simulink model "SuR_Projekt_Wegpunkt_v3"  (R2023a)
settings: Solver=FixedStepDiscrete  StartTime=0.0  StopTime=inf  FixedStep=0.1  RelTol=1e-3  EnableMultiTasking=on
libraries: quarc_library x6
settings Model: ExtModeTrigDuration=10000  Creator=Student  LastModifiedBy=Student
settings SolverCC: AlgebraicLoopSolver=TrustRegion  PositivePriorityOrder=on
settings DataIOCC: ReturnWorkspaceOutputs=off
settings DebuggingCC: UnconnectedInputMsg=warning  UnconnectedOutputMsg=warning  UnconnectedLineMsg=warning  ArithmeticOperatorsInVariantConditions=warning
settings ModelReferenceCC: EnableRefExpFcnMdlSchedulingChecks=on
settings SFSimCC: SimUseLocalCustomCode=off  CustomCodeUndefinedFunction=UseInterfaceOnly
settings RTWCC: Description=QUARC Win64 Target Using Toolchain  SystemTargetFile=quarc_win64.tlc  TemplateMakefile=quarc_default_tmf  RTWUseLocalCustomCode=off  Toolchain=QUARC win64 | nmake (64-bit Windows)  BuildConfiguration=Faster Runs
settings CodeAppCC: StateflowObjectComments=on
settings STFCustomTargetCC: SystemTargetFile=quarc_win64.tlc
settings GRTTargetCC: ParMdlRefBuildCompliant=off  CompOptLevelCompliant=off  CombineOutputUpdateFcns=off  MatFileLogging=off  CPPClassGenCompliant=off  GRTInterface=on  ExtMode=on  ExtModeMexFile=quarc_comm
settings ConfigComp: CovMetricSettings=dswe

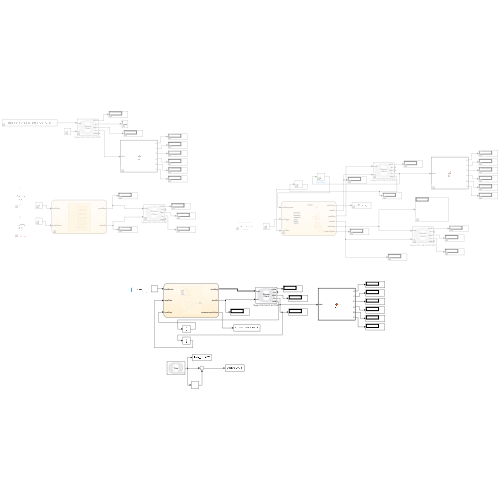
[thumbnail: Simulink's stored preview of the top-level diagram]
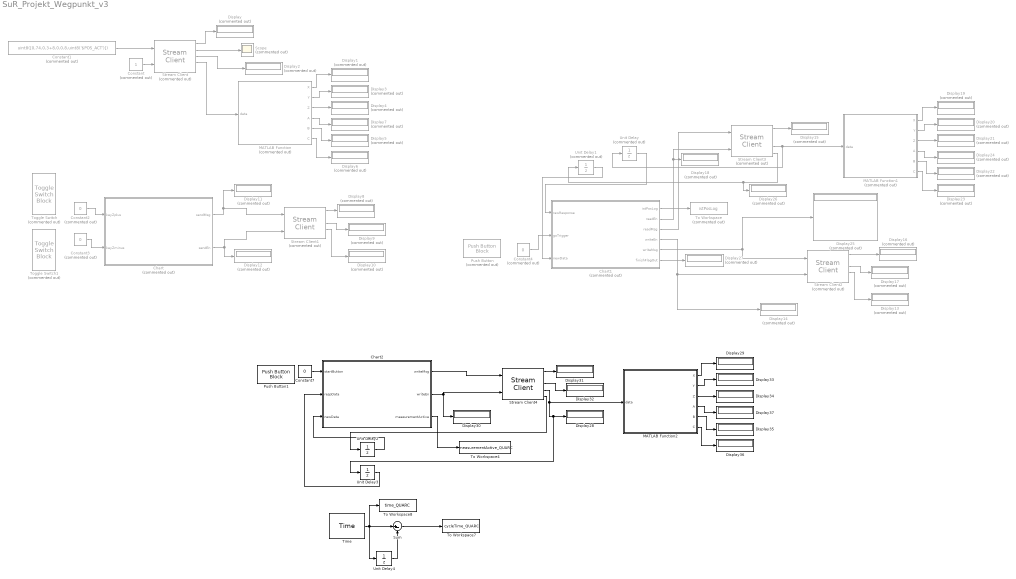
== system SuR_Projekt_Wegpunkt_v3 ==
  Chart : Stateflow chart  Commented=on  TreatAsAtomicUnit=on
  Chart1 : Stateflow chart  Commented=on  TreatAsAtomicUnit=on
  Chart2 : Stateflow chart  TreatAsAtomicUnit=on
  Constant : Constant  Commented=on
  Constant1 : Constant  Commented=on  Value=uint8([0,74,0,3+8,0,0,8,uint8('$POS_ACT')])  OutDataTypeStr=uint8
  Constant2 : Constant  Commented=on  Value=0  OutDataTypeStr=boolean
  Constant3 : Constant  Commented=on  Value=0  OutDataTypeStr=boolean
  Constant4 : Constant  Commented=on  Value=0  OutDataTypeStr=boolean
  Constant7 : Constant  Value=0
  Display{,1..27} (28 alike) : Display  Commented=on
  Display{28..37} (10 alike) : Display
  MATLAB Function : MATLAB Function  Commented=on  TreatAsAtomicUnit=on
  MATLAB Function1 : MATLAB Function  Commented=on  TreatAsAtomicUnit=on
  MATLAB Function2 : MATLAB Function  TreatAsAtomicUnit=on
  Push Button : PushButtonBlock  Commented=on  OffValue=0.000000
  Push Button1 : PushButtonBlock  OffValue=0.000000
  Scope : Scope  Commented=on
  Stream Client : quarc_library/Communications/Basic/Stream Client  Commented=on  uri_source=Specify via dialog (do not evaluate)  uri=tcpip://192.168.41.64:7000  send_buffer_size=1460  receive_buffer_size=1460  byte_order=little endian (Intel - LSB first)  optimization=Minimum latency  send_options=Send all data  receive_options=Receive all data  default_value=[uint8(0);uint8(0);uint8(0);uint8(0);uint8(0);uint8(0);uint8(0);uint8(0);uint8(0);uint8(0);uint8(0);uint8(0);uint8(0);uint8(0);uint8(0);uint8(0);uint8(0);uint8(0);uint8(0);uint8(0);uint8(0);uint8(0);uint8(0);uint8(0);uint8(0);uint8(0);uint8(0);uint8(0);uint8(0);uint8(0);uint8(0);uint8(0);uint8(0);uint8(0);uint8(0);uint8(0);uint8(0);uint8(0);uint8(0);uint8(0);uint8(0);uint8(0);uint8(0);uint8(0);uint8(0);uint8(0);uint8(0);uint8(0);uint8(0);uint8(0);uint8(0);uint8(0);uint8(0);uint8(0);uint8(0);uint8(0);uint8(0);uint8(0);uint8(0);uint8(0);uint8(0);uint8(0);uint8(0);uint8(0);uint8(0);uint8(0);uint8(0);uint8(0);uint8(0);uint8(0);uint8(0);uint8(0);uint8(0);uint8(0);uint8(0);uint8(0);uint8(0);uint8(0);uint8(0);uint8(0);uint8(0);uint8(0);uint8(0);uint8(0);uint8(0);uint8(0);uint8(0);uint8(0);uint8(0);uint8(0);uint8(0);uint8(0);uint8(0);uint8(0);uint8(0);uint8(0);uint8(0);uint8(0);uint8(0);uint8(0);uint8(0);uint8(0);uint8(0);uint8(0);uint8(0);uint8(0);uint8(0);uint8(0);uint8(0);uint8(0);uint8(0);uint8(0);uint8(0);uint8(0);uint8(0);uint8(0);uint8(0);uint8(0);uint8(0);uint8(0);uint8(0);uint8(0);uint8(0);uint8(0);uint8(0);uint8(0);uint8(0);uint8(0);uint8(0);uint8(0);uint8(0);uint8(0);uint8(0);uint8(0);uint8(0);uint8(0);uint8(0);uint8(0);uint8(0);uint8(0);uint8(0);uint8(0);uint8(0);uint8(0);uint8(0);uint8(0);uint8(0);uint8(0);uint8(0);uint8(0);uint8(0);uint8(0);uint8(0);uint8(0);uint8(0);uint8(0);uint8(0);uint8(0);uint8(0);uint8(0);uint8(0);uint8(0);uint8(0);uint8(0);uint8(0);uint8(0);uint8(0);uint8(0);uint8(0);uint8(0);uint8(0);uint8(0);uint8(0);uint8(0);uint8(0);uint8(0);uint8(0);uint8(0);uint8(0);uint8(0);uint8(0);uint8(0);uint8(0);uint8(0);uint8(0);uint8(0);uint8(0);uint8(0);uint8(0);uint8(0);uint8(0);uint8(0);uint8(0);uint8(0);uint8(0);uint8(0);uint8(0);uint8(0);uint8(0);uint8(0);uint8(0);uint8(0);uint8(0);uint8(0);uint8(0);uint8(0);uint8(0);uint8(0);uint8(0);uint8(0);uint8(0);uint8(0);uint8(0);uint8(0);uint8(0);uint8(0);uint8(0);uint8(0);uint8(0);uint8(0);uint8(0);uint8(0);uint8(0);uint8(0);uint8(0);uint8(0);uint8(0);uint8(0);uint8(0);uint8(0);uint8(0);uint8(0);uint8(0);uint8(0);uint8(0);uint8(0);uint8(0);uint8(0);uint8(0);uint8(0);uint8(0);uint8(0);uint8(0);uint8(0);uint8(0);uint8(0);uint8(0);uint8(0);uint8(0);uint8(0);uint8(0);uint8(0);uint8(0);uint8(0);uint8(0);uint8(0)]  sample_time=qc_get_step_size  active=off  implementation=Use blocking I/O in a separate thread  send_fifo_size=1000  receive_fifo_size=1000  send_priority=0  receive_priority=0  send_dimensions=off  receive_dimensions=off  max_dimensions=-1  data_type=uint8  type_expr=BusObject
      settings: AttributesFormatString="\"tcpip://192.168.41.64:7000\""
  Stream Client1 : quarc_library/Communications/Basic/Stream Client  Commented=on  uri_source=Specify via dialog (do not evaluate)  uri=tcpip://192.168.41.64:7000  send_buffer_size=1460  receive_buffer_size=1460  byte_order=little endian (Intel - LSB first)  optimization=Minimum latency  send_options=Send all data  receive_options=Receive all data  default_value=zeros(256,1,'uint8')  sample_time=qc_get_step_size  active=off  implementation=Use blocking I/O in a separate thread  send_fifo_size=1000  receive_fifo_size=1000  send_priority=0  receive_priority=0  send_dimensions=off  receive_dimensions=off  max_dimensions=-1  data_type=uint8  type_expr=BusObject
      settings: AttributesFormatString="\"tcpip://192.168.41.64:7000\""
  Stream Client2 : quarc_library/Communications/Basic/Stream Client  Commented=on  uri_source=Specify via dialog (do not evaluate)  uri=tcpip://192.168.41.64:7000  send_buffer_size=1460  receive_buffer_size=1460  byte_order=little endian (Intel - LSB first)  optimization=Minimum latency  send_options=Send all data  receive_options=Receive all data  default_value=zeros(256,1,'uint8')  sample_time=qc_get_step_size  active=off  implementation=Use blocking I/O in a separate thread  send_fifo_size=1000  receive_fifo_size=1000  send_priority=0  receive_priority=0  send_dimensions=off  receive_dimensions=off  max_dimensions=-1  data_type=uint8  type_expr=BusObject
      settings: AttributesFormatString="\"tcpip://192.168.41.64:7000\""
  Stream Client3 : quarc_library/Communications/Basic/Stream Client  Commented=on  uri_source=Specify via dialog (do not evaluate)  uri=tcpip://192.168.41.64:7000  send_buffer_size=1460  receive_buffer_size=1460  byte_order=little endian (Intel - LSB first)  optimization=Minimum latency  send_options=Send all data  receive_options=Receive all data  default_value=zeros(256,1,'uint8')  sample_time=qc_get_step_size  active=off  implementation=Use blocking I/O in a separate thread  send_fifo_size=1000  receive_fifo_size=1000  send_priority=0  receive_priority=0  send_dimensions=off  receive_dimensions=off  max_dimensions=-1  data_type=uint8  type_expr=BusObject
      settings: AttributesFormatString="\"tcpip://192.168.41.64:7000\""
  Stream Client4 : quarc_library/Communications/Basic/Stream Client  uri_source=Specify via dialog (do not evaluate)  uri=tcpip://192.168.41.64:7000  send_buffer_size=1460  receive_buffer_size=1460  byte_order=little endian (Intel - LSB first)  optimization=Minimum latency  send_options=Send all data  receive_options=Receive all data  default_value=zeros(256,1,'uint8')  sample_time=qc_get_step_size  active=off  implementation=Use blocking I/O in a separate thread  send_fifo_size=1000  receive_fifo_size=1000  send_priority=0  receive_priority=0  send_dimensions=off  receive_dimensions=off  max_dimensions=-1  data_type=uint8  type_expr=BusObject
      settings: AttributesFormatString="\"tcpip://192.168.41.64:7000\""
  Sum : Sum  Inputs=|+-
  Time : quarc_library/Sources/Time/Time  time_source=Wall clock  sample_time=qc_get_step_size
  To Workspace : ToWorkspace  Commented=on  VariableName=istPosLog  SampleTime=-1
  To Workspace4 : ToWorkspace  VariableName=measurementActive_QUARC  SaveFormat=Structure With Time  SampleTime=-1
  To Workspace7 : ToWorkspace  VariableName=cycleTime_QUARC  SaveFormat=Structure With Time  SampleTime=-1
  To Workspace8 : ToWorkspace  VariableName=time_QUARC  SaveFormat=Structure With Time  SampleTime=-1
  Toggle Switch : ToggleSwitchBlock  Commented=on
      settings: Values={{'Off', 'On'}, [0 1]}
  Toggle Switch1 : ToggleSwitchBlock  Commented=on
      settings: Values={{'Off', 'On'}, [0 1]}
  Unit Delay : UnitDelay  Commented=on  InitialCondition=uint8(zeros(1,256))  SampleTime=-1  HasFrameUpgradeWarning=on
  Unit Delay1 : UnitDelay  Commented=on  InitialCondition=uint8(zeros(1,1))  SampleTime=-1  HasFrameUpgradeWarning=on
  Unit Delay2 : UnitDelay  InitialCondition=uint8(zeros(1,1))  SampleTime=-1  HasFrameUpgradeWarning=on
  Unit Delay3 : UnitDelay  InitialCondition=uint8(zeros(1,256))  SampleTime=-1  HasFrameUpgradeWarning=on
  Unit Delay4 : UnitDelay  SampleTime=-1  HasFrameUpgradeWarning=on
  wires:
  Stream Client/1 -> Display/1
  Stream Client/2 -> Scope/1
  Constant1/1 -> Stream Client/1
  Stream Client/4 -> MATLAB Function/1(data)
  Stream Client/3 -> Display2/1
  MATLAB Function/1(X) -> Display1/1
  MATLAB Function/2(Y) -> Display3/1
  MATLAB Function/3(Z) -> Display4/1
  MATLAB Function/4(A) -> Display7/1
  MATLAB Function/5(B) -> Display5/1
  MATLAB Function/6(C) -> Display6/1
  Stream Client1/1 -> Display8/1
  Constant/1 -> Stream Client/2
  Chart/1(sendMsg) -> Display11/1, Stream Client1/1
  Chart/2(sendEn) -> Stream Client1/2, Display12/1
  Constant3/1 -> Chart/2(keyZminus)
  Stream Client1/3 -> Display9/1
  Stream Client1/4 -> Display10/1
  Constant2/1 -> Chart/1(keyZplus)
  Stream Client2/4 -> Display13/1
  Stream Client2/1 -> Display16/1
  Stream Client2/3 -> Display17/1
  Constant4/1 -> Chart1/2(goTrigger)
  Chart1/5(writeMsg) -> Stream Client2/1, Display25/1
  Chart1/4(writeEn) -> Display14/1, Stream Client2/2
  Chart1/3(readMsg) -> Stream Client3/1
  Chart1/2(readEn) -> Stream Client3/2, Display18/1
  Chart1/1(istPosLog) -> To Workspace/1
  Stream Client3/1 -> Display15/1
  Stream Client3/4 -> MATLAB Function1/1(data), Unit Delay/1
  Unit Delay/1 -> Chart1/1(rawResponse)
  MATLAB Function1/4(A) -> Display24/1
  MATLAB Function1/6(C) -> Display23/1
  MATLAB Function1/3(Z) -> Display21/1
  MATLAB Function1/2(Y) -> Display20/1
  MATLAB Function1/5(B) -> Display22/1
  MATLAB Function1/1(X) -> Display19/1
  Chart1/6(finishFlagOut) -> Display27/1
  Unit Delay1/1 -> Chart1/3(newData)
  Stream Client3/5 -> Display26/1, Unit Delay1/1
  Stream Client4/3 -> Display32/1
  Stream Client4/4 -> MATLAB Function2/1(data), Unit Delay3/1, Display28/1
  Stream Client4/1 -> Display31/1
  Constant7/1 -> Chart2/1(startButton)
  Chart2/2(writeEn) -> Display30/1, Stream Client4/2
  Chart2/1(writeMsg) -> Stream Client4/1
  Time/1 -> To Workspace8/1, Unit Delay4/1, Sum/1
  Unit Delay4/1 -> Sum/2
  Sum/1 -> To Workspace7/1
  Chart2/3(measurementActive) -> To Workspace4/1
  MATLAB Function2/4(A) -> Display37/1
  MATLAB Function2/6(C) -> Display36/1
  MATLAB Function2/1(X) -> Display29/1
  MATLAB Function2/2(Y) -> Display33/1
  MATLAB Function2/3(Z) -> Display34/1
  MATLAB Function2/5(B) -> Display35/1
  Stream Client4/5 -> Unit Delay2/1
  Unit Delay2/1 -> Chart2/3(newData)
  Unit Delay3/1 -> Chart2/2(respData)

== stateflow chart SuR_Projekt_Wegpunkt_v3/Chart1 ==
  state INIT
    entry:
    writeMsg = buildActPrepMsg();   % ACTFLAG=TRUE, PROGVAR=1, ENDPROG=TRUE
    writeEn = true;
  state SEND_WP1
    entry:
    writeMsg = buildWriteFrame(wpMatrix, movemodeArr, velArr, gripArr, 1, 1);
    writeEn = true;
  state SEND_WP2
    entry:
    writeMsg = buildWriteFrame(wpMatrix, movemodeArr, velArr, gripArr, 2, 2);
    writeEn = true;
  state WAIT_GO
    entry:
    writeEn = false;
  state START_WAIT
    entry:
    writeEn = false;
  state START
    entry:
    writeMsg = buildStartMsg();   % STARTVAR = TRUE
    writeEn = true;
  state POLL_SEND
    entry:
    readEn = false;
    finishFlag = false;
    readMsg = buildReadFrame(actMove);
    readEn = true;
  state POLL_WAIT
    exit:
    readEn = false;
  state PROCESS_RESPONSE
    entry:
    [finishFlag, istPosLog] = parseResponse(rawResponse, actMove);
    finishFlagOut = finishFlag;
  state ADVANCE
    entry:
    readEn = false;
    writeEn = false;
  state SEND_NEXT
    entry:
    writeEn = false;
    counter = counter +1;
    if actMove ==1
    bufIdx = 1;
    actMove = 2;
    else
    bufIdx = 2;
    actMove = 1;
    end
    writeMsg = buildWriteFrame(wpMatrix, movemodeArr, velArr, gripArr, counter, bufIdx);
    writeEn = true;
    finishFlag = false;
  state SEND_END
    entry:
    readEn = false;
    writeEn = false;
    writeMsg = buildEndProgMsg();
    writeEn = true;
    endSent = true;
  state DONE
    entry:
    writeEn = false;
    readEn = false;
  (default) -> INIT
  INIT -> SEND_WP1 : after(10,tick)
  SEND_WP1 -> SEND_WP2 : after(10,tick)
  SEND_WP2 -> WAIT_GO : after(1,tick)
  WAIT_GO -> START : [goTrigger]
  START -> START_WAIT : after(1,tick)
  START_WAIT -> POLL_SEND : after(10,tick)
  POLL_SEND -> POLL_WAIT : after(1,tick)
  SEND_NEXT -> POLL_SEND : after(1, tick)
  PROCESS_RESPONSE -> POLL_SEND [order 1] : [~finishFlag]
  POLL_WAIT -> PROCESS_RESPONSE : [newData]
  PROCESS_RESPONSE -> ADVANCE [order 2] : [finishFlag]
  ADVANCE -> SEND_NEXT [order 1] : [counter < 5]
  ADVANCE -> SEND_END [order 2] : [counter >= 5]
  SEND_END -> DONE : after(1, tick)
  data: msg function_output; wp function_input; modeArr function_input; velArr function_input; gripArr function_input; wpIdx function_input; bufIdx function_input; msg function_output size=[1 160]; bufIdx function_input; msg function_output; resp function_input; bufIdx function_input; finish function_output; posLog function_output; msg function_output size=[1 160]; msg function_output size=[1 160]; msg function_output size=[1 160]; actMove local uint8 =1; finishFlag local boolean =false; endSent local boolean =false; counter local double =2; istPosLog output double size=[1 8]; readEn output boolean size=[1]; readMsg output uint8 size=[1 29]; writeEn output boolean size=[1]; writeMsg output uint8 size=[1 160]; rawResponse input uint8 size=[1 256]; goTrigger input boolean size=[1]; wpMatrix constant double size=[5 8] =[426.9750, 54.0223, 574.0360, 90.0000, 89.0000, 90.0000, 2, 35; 420.1710, -93.1800, 574.0360, 70.2850, 89.0000, 90.0000, 2, 42; 466.6860, -109.8400, 443.9820, 156.8940, 72.8388, 176.7590, 2, 42; 477.7830, 39.8285, 443.9820, 174.9040, 72.8388, 176.7590, 2, 42; 426.9750, 54.0223, 574.0360, 90.0000, 89.0000, 90.0000, 2, 42]; movemodeArr constant double size=[1 5] =[1,1,1,1,1]; velArr constant double size=[1 5] =[15,15,15,15,15]; gripArr constant double size=[1 5] =[1,1,1,1,1]; bufIdx local uint8 =1; finishFlagOut output; newData input boolean size=[1]
  function msg = buildActFlagTrueMsg:
    | function msg = buildActFlagTrueMsg()
    | 
    | msg = uint8([0,60,0,16,1,0,7,uint8('ACTFLAG'),0,4,uint8('TRUE')]);
    | 
    | end
  function msg = buildWriteFrame(wp, modeArr, velArr, gripArr, wpIdx, bufIdx):
    | function msg = buildWriteFrame(wp, modeArr, velArr, gripArr, wpIdx, bufIdx)
    | 
    | x = wp(wpIdx,1);
    | y = wp(wpIdx,2);
    | z = wp(wpIdx,3);
    | a = wp(wpIdx,4);
    | b = wp(wpIdx,5);
    | c = wp(wpIdx,6);
    | 
    | s = int32(wp(wpIdx,7));
    | t = int32(wp(wpIdx,8));
    | 
    | % KUKA E6POS String
    | % Kein + und keine führenden Nullen
    | posval_char = sprintf( ...
    |     '{POS: X %.1f,Y %.1f,Z %.1f,A %.1f,B %.1f,C %.1f,S %d,T %d}', ...
    |     x,y,z,a,b,c,s,t);
    | 
    | posval = uint8(posval_char);
    | 
    | % Weitere Werte
    | velval_char  = sprintf('%.1f',velArr(wpIdx));
    | modval_char  = sprintf('%d',int32(modeArr(wpIdx)));
    | gripval_char = sprintf('%d',int32(gripArr(wpIdx)));
    | 
    | velval  = uint8(velval_char);
    | modval  = uint8(modval_char);
    | gripval = uint8(gripval_char);
    | 
    | 
    | if bufIdx == 1
    | 
    |     modmsg = uint8([ ...
    |         0,11, ...
    |         0,3+9+2+length(modval), ...
    |         1, ...
    |         0,9, ...
    |         uint8('MOVEMODE1'), ...
    |         0,length(modval), ...
    |         modval]);
    | 
    |     posmsg = uint8([ ...
    |         0,13, ...
    |         0,3+8+2+length(posval), ...
    |         1, ...
    |         0,8, ...
    |         uint8('MAT_POS1'), ...
    |         0,length(posval), ...
    |         posval]);
    | 
    |     grpmsg = uint8([ ...
    |         0,17, ...
    |         0,3+4+2+length(gripval), ...
    |         1, ...
    |         0,4, ...
    |         uint8('GRP1'), ...
    |         0,length(gripval), ...
    |         gripval]);
    | 
    |     velmsg = uint8([ ...
    |         0,15, ...
    |         0,3+4+length(velval), ...
    |         1, ...
    |         0,4, ...
    |         uint8('VEL1'), ...
    |         0,length(velval), ...
    |         velval]);
    | 
    | else
    | 
    |     modmsg = uint8([ ...
    |         0,22, ...
    |         0,3+9+2+length(modval), ...
    |         1, ...
    |         0,9, ...
    |         uint8('MOVEMODE2'), ...
    |         0,length(modval), ...
    |         modval]);
    | 
    |     posmsg = uint8([ ...
    |         0,42, ...
    |         0,3+8+2+length(posval), ...
    |         1, ...
    |         0,8, ...
    |         uint8('MAT_POS2'), ...
    |         0,length(posval), ...
    |         posval]);
    | 
    |     grpmsg = uint8([ ...
    |         0,82, ...
    |         0,3+4+2+length(gripval), ...
    |         1, ...
    |         0,4, ...
    |         uint8('GRP2'), ...
    |         0,length(gripval), ...
    |         gripval]);
    | 
    |     velmsg = uint8([ ...
    |         0,62, ...
    |         0,3+4+length(velval), ...
    |         1, ...
    |         0,4, ...
    |         uint8('VEL2'), ...
    |         0,length(velval), ...
    |         velval]);
    | 
    | end
    | 
    | msg = [modmsg,posmsg,grpmsg,velmsg];
    | 
    | end
  function msg = buildReadFrame(bufIdx):
    | function msg = buildReadFrame(bufIdx)
    |     readposmsg = uint8([0,74,0,3+8,0,0,8,uint8('$POS_ACT')]);
    |     if(bufIdx == 1)
    |         readmsg = uint8([0,90,0,3+7,0,0,7,uint8('FINISH1')]);
    |     else
    |         readmsg = uint8([0,91,0,3+7,0,0,7,uint8('FINISH2')]);
    |     end
    |     msg = [readmsg, readposmsg];
    | end
  function [finish, posLog] = parseResponse(resp, bufIdx):
    | function [finish, posLog] = parseResponse(resp, bufIdx)
    | 
    | % -------------------------------------------------------------
    | % Robuster KUKAVARPROXY Parser
    | % Sucht FINISH1/FINISH2 und $POS_ACT innerhalb des gesamten
    | % empfangenen Puffers, statt feste Bytepositionen vorauszusetzen.
    | % -------------------------------------------------------------
    | 
    | finish = false;
    | posLog = zeros(1,8);
    | 
    | r = uint8(resp(:)');
    | N = numel(r);
    | 
    | if N < 2
    |     return;
    | end
    | 
    | expectedId = uint8(89 + double(bufIdx));   % 90 = FINISH1, 91 = FINISH2
    | 
    | 
    | %% =============================================================
    | % 1. FINISH-Antwort im gesamten Buffer suchen
    | % =============================================================
    | 
    | for i = 1:(N-1)
    | 
    |     % Beginn einer KVP-Antwort:
    |     % Bytefolge [0 90] bzw. [0 91]
    |     if r(i) == 0 && r(i+1) == expectedId
    | 
    |         % Genug Bytes für Header?
    |         if i + 6 <= N
    | 
    |             valueLen = double(r(i+6));
    | 
    |             % Plausible Länge prüfen
    |             if valueLen == 4 || valueLen == 5
    | 
    |                 % Antwortwert kann etwas später im Frame liegen.
    |                 % Deshalb nicht blind feste Position verwenden,
    |                 % sondern in einem kleinen Bereich nach ASCII TRUE/FALSE suchen.
    | 
    |                 searchEnd = min(N, i + 25);
    | 
    |                 % ---- TRUE suchen ----
    |                 for k = i:min(searchEnd-3, N-3)
    | 
    |                     if r(k)   == uint8('T') && ...
    |                        r(k+1) == uint8('R') && ...
    |                        r(k+2) == uint8('U') && ...
    |                        r(k+3) == uint8('E')
    | 
    |                         finish = true;
    |                         break;
    |                     end
    |                 end
    | 
    |                 if finish
    |                     break;
    |                 end
    | 
    |                 % FALSE bedeutet explizit: Bewegung noch nicht fertig
    |                 if valueLen == 5
    |                     finish = false;
    |                 end
    |             end
    |         end
    |     end
    | end
    | 
    | 
    | %% =============================================================
    | % 2. POS-Struktur im gesamten Buffer suchen
    | %
    | % Wir verlassen uns NICHT darauf, dass $POS_ACT bei Byte 16/17
    | % beginnt. Stattdessen suchen wir direkt nach "{POS:"
    | % =============================================================
    | 
    | posBegin = 0;
    | 
    | for i = 1:(N-4)
    | 
    |     if r(i)   == uint8('{') && ...
    |        r(i+1) == uint8('P') && ...
    |        r(i+2) == uint8('O') && ...
    |        r(i+3) == uint8('S') && ...
    |        r(i+4) == uint8(':')
    | 
    |         posBegin = i;
    |         break;
    |     end
    | end
    | 
    | % Noch keine vollständige Positionsantwort vorhanden
    | if posBegin == 0
    |     return;
    | end
    | 
    | 
    | %% =============================================================
    | % 3. Ende der POS-Struktur suchen
    | % =============================================================
    | 
    | posEnd = 0;
    | 
    | for i = posBegin:N
    |     if r(i) == uint8('}')
    |         posEnd = i;
    |         break;
    |     end
    | end
    | 
    | if posEnd == 0
    |     return;
    | end
    | 
    | p = r(posBegin:posEnd);
    | n = numel(p);
    | 
    | 
    | %% =============================================================
    | % 4. Marker X Y Z A B C S T finden
    | % =============================================================
    | 
    | markers = uint8(['X','Y','Z','A','B','C','S','T']);
    | startind = zeros(1,8);
    | 
    | for m = 1:8
    | 
    |     idx = 0;
    | 
    |     if m == 7
    |         % S: letztes S nehmen, damit nicht das S aus "POS" erkannt wird
    |         for k = n:-1:1
    |             if p(k) == markers(m)
    |                 idx = k;
    |                 break;
    |             end
    |         end
    | 
    |     else
    |         for k = 1:n
    |             if p(k) == markers(m)
    |                 idx = k;
    |                 break;
    |             end
    |         end
    |     end
    | 
    |     if idx == 0
    |         return;
    |     end
    | 
    |     % Format z.B. "X 426.9"
    |     startind(m) = idx + 2;
    | end
    | 
    | 
    | %% =============================================================
    | % 5. Trennzeichen bestimmen
    | % =============================================================
    | 
    | commaIdx = zeros(1,7);
    | c = 0;
    | 
    | for k = 1:n
    | 
    |     if p(k) == uint8(',')
    | 
    |         c = c + 1;
    | 
    |         if c <= 7
    |             commaIdx(c) = k;
    |         end
    |     end
    | end
    | 
    | if c < 7
    |     return;
    | end
    | 
    | braceIdx = n;    % p endet bereits bei }
    | 
    | 
    | %% =============================================================
    | % 6. Werte konvertieren
    | % =============================================================
    | 
    | endind = zeros(1,8);
    | 
    | endind(1:7) = commaIdx - 1;
    | endind(8)   = braceIdx - 1;
    | 
    | tmp = zeros(1,8);
    | 
    | for m = 1:8
    | 
    |     if startind(m) > endind(m)
    |         return;
    |     end
    | 
    |     txt = char(p(startind(m):endind(m)));
    | 
    |     val = real(str2double(txt));
    | 
    |     if isnan(val)
    |         return;
    |     end
    | 
    |     tmp(m) = val;
    | end
    | 
    | posLog = tmp;
    | 
    | end
  function msg = buildActPrepMsg:
    | function msg = buildActPrepMsg()
    |     actmsg   = uint8([0,60,0,3+7+6,1,0,7,uint8('ACTFLAG'),0,4,uint8('TRUE')]);
    |     progmsg  = uint8([0,30,0,3+7+3,1,0,7,uint8('PROGVAR'),0,4,uint8('1')]);
    |     endmsg   = uint8([0,20,0,3+7+6,1,0,7,uint8('ENDPROG'),0,4,uint8('TRUE')]);
    |     msg = [actmsg, progmsg, endmsg];   % keine Auffüllung mehr nötig
    | end
  function msg = buildStartMsg:
    | function msg = buildStartMsg()
    |     startmsg = uint8([0,10,0,3+8+6,1,0,8,uint8('STARTVAR'),0,4,uint8('TRUE')]);
    |     msg = startmsg;
    | end
  function msg = buildEndProgMsg:
    | function msg = buildEndProgMsg()
    |     endmsg = uint8([0,20,0,3+7+6,1,0,7,uint8('ENDPROG'),0,4,uint8('TRUE')]);
    |     msg = endmsg;
    | end

== matlab function SuR_Projekt_Wegpunkt_v3/MATLAB Function ==
  data: data input; X output; Y output; Z output; A output; B output; C output
function [X,Y,Z,A,B,C] = fcn(data)

% Standardwerte
X = NaN;
Y = NaN;
Z = NaN;
A = NaN;
B = NaN;
C = NaN;

% Empfangsdaten in einen Vektor umwandeln
data = data(:);

% Positionen suchen
ix = find(data == 88, 1, 'first');   % X
iy = find(data == 89, 1, 'first');   % Y
iz = find(data == 90, 1, 'first');   % Z
ia = find(data == 65, 1, 'first');   % A
ib = find(data == 66, 1, 'first');   % B
ic = find(data == 67, 1, 'first');   % C

% Zahlen auslesen
if ~isempty(ix)
    X = parseNumber(data, ix + 1);
end

if ~isempty(iy)
    Y = parseNumber(data, iy + 1);
end

if ~isempty(iz)
    Z = parseNumber(data, iz + 1);
end

if ~isempty(ia)
    A = parseNumber(data, ia + 1);
end

if ~isempty(ib)
    B = parseNumber(data, ib + 1);
end

if ~isempty(ic)
    C = parseNumber(data, ic + 1);
end

end


function value = parseNumber(data, startIndex)

value = 0;

n = numel(data);
idx = startIndex;

% Sicherstellen, dass idx ein Skalar ist
idx = idx(1);

% Leerzeichen überspringen
while idx <= n
    if data(idx) ~= 32
        break;
    end
    idx = idx + 1;
end

% Vorzeichen
sgn = 1;

if idx <= n
    if data(idx) == 45       % '-'
        sgn = -1;
        idx = idx + 1;
    elseif data(idx) == 43   % '+'
        idx = idx + 1;
    end
end

% Ganzzahlteil
while idx <= n
    if data(idx) < 48 || data(idx) > 57
        break;
    end

    value = value * 10 + double(data(idx) - 48);
    idx = idx + 1;
end

% Nachkommastellen
if idx <= n && data(idx) == 46       % '.'
    idx = idx + 1;

    factor = 0.1;

    while idx <= n
        if data(idx) < 48 || data(idx) > 57
            break;
        end

        value = value + double(data(idx) - 48) * factor;
        factor = factor * 0.1;
        idx = idx + 1;
    end
end

value = sgn * value;

end

== stateflow chart SuR_Projekt_Wegpunkt_v3/Chart ==
  state Superstate
    during:
    riseZplus  = keyZplus  && ~prevZplus;
    riseZminus = keyZminus && ~prevZminus;
    fallActive = (activeKey==6 && ~keyZplus) || (activeKey==5 && ~keyZminus);
    state IDLE
      entry:
      sendEn = false;
    state SEND_ACT_ON
      entry:
      sendMsg = msgActOn;
      sendEn = true;
    state SEND_MOVE
      entry:
      if(activeKey == 6)
      sendMsg = msgKeyZplus;
      else
      sendMsg = msgKeyZminus;
      end
      sendEn = true;
    state HOLD
      entry:
      sendEn = false;
    state SEND_KEYFLAG0
      entry:
      sendMsg = msgKey0;
      sendEn = true;
    state SEND_ACT_OFF
      entry:
      sendMsg = msgActOff;
      sendEn = true;
      activeKey = 0;
    (default) -> IDLE
    SEND_ACT_OFF -> IDLE
    IDLE -> SEND_ACT_ON [order 2] : [riseZminus]/{activeKey = 5;}
    IDLE -> SEND_ACT_ON [order 1] : [riseZplus]/{activeKey = 6;}
    SEND_ACT_ON -> SEND_MOVE
    SEND_MOVE -> HOLD
    HOLD -> SEND_KEYFLAG0 : [fallActive]
    SEND_KEYFLAG0 -> SEND_ACT_OFF
  data: sendMsg output uint8 size=[1 21]; sendEn output boolean size=[1]; msgKeyZminus constant uint8 size=[1 21] =uint8([0,5,0,14,1,0,7,uint8('KEYFLAG'),0,2,uint8('05'),0,0,0]); msgKeyZplus constant uint8 size=[1 21] =uint8([0,6,0,14,1,0,7,uint8('KEYFLAG'),0,2,uint8('06'),0,0,0]); msgKey0 constant uint8 size=[1 21] =uint8([0,21,0,13,1,0,7,uint8('KEYFLAG'),0,1,uint8('0'),0,0,0,0]); msgActOn constant uint8 size=[1 21] =uint8([0,60,0,16,1,0,7,uint8('ACTFLAG'),0,4,uint8('TRUE'),0]); msgActOff constant uint8 size=[1 21] =uint8([0,60,0,17,1,0,7,uint8('ACTFLAG'),0,5,uint8('FALSE')]); activeKey local uint8; prevZplus local boolean size=[1]; prevZminus local boolean size=[1]; keyZplus input boolean size=[1]; keyZminus input boolean size=[1]; fallActive local boolean size=[1]; riseZminus local boolean size=[1]; riseZplus local boolean size=[1]

== matlab function SuR_Projekt_Wegpunkt_v3/MATLAB Function1 ==
  data: data input; X output; Y output; Z output; A output; B output; C output
function [X,Y,Z,A,B,C] = fcn(data)

% Standardwerte
X = NaN;
Y = NaN;
Z = NaN;
A = NaN;
B = NaN;
C = NaN;

% Empfangsdaten in einen Vektor umwandeln
data = data(:);

% Positionen suchen
ix = find(data == 88, 1, 'first');   % X
iy = find(data == 89, 1, 'first');   % Y
iz = find(data == 90, 1, 'first');   % Z
ia = find(data == 65, 1, 'first');   % A
ib = find(data == 66, 1, 'first');   % B
ic = find(data == 67, 1, 'first');   % C

% Zahlen auslesen
if ~isempty(ix)
    X = parseNumber(data, ix + 1);
end

if ~isempty(iy)
    Y = parseNumber(data, iy + 1);
end

if ~isempty(iz)
    Z = parseNumber(data, iz + 1);
end

if ~isempty(ia)
    A = parseNumber(data, ia + 1);
end

if ~isempty(ib)
    B = parseNumber(data, ib + 1);
end

if ~isempty(ic)
    C = parseNumber(data, ic + 1);
end

end


function value = parseNumber(data, startIndex)

value = 0;

n = numel(data);
idx = startIndex;

% Sicherstellen, dass idx ein Skalar ist
idx = idx(1);

% Leerzeichen überspringen
while idx <= n
    if data(idx) ~= 32
        break;
    end
    idx = idx + 1;
end

% Vorzeichen
sgn = 1;

if idx <= n
    if data(idx) == 45       % '-'
        sgn = -1;
        idx = idx + 1;
    elseif data(idx) == 43   % '+'
        idx = idx + 1;
    end
end

% Ganzzahlteil
while idx <= n
    if data(idx) < 48 || data(idx) > 57
        break;
    end

    value = value * 10 + double(data(idx) - 48);
    idx = idx + 1;
end

% Nachkommastellen
if idx <= n && data(idx) == 46       % '.'
    idx = idx + 1;

    factor = 0.1;

    while idx <= n
        if data(idx) < 48 || data(idx) > 57
            break;
        end

        value = value + double(data(idx) - 48) * factor;
        factor = factor * 0.1;
        idx = idx + 1;
    end
end

value = sgn * value;

end

== stateflow chart SuR_Projekt_Wegpunkt_v3/Chart2 ==
  state Superstate
    state IDLE
      entry:
      writeEn = false;
      measurementActive = false;
    state INIT_END
      entry:
      writeMsg = buildEndTrueMsg();
      writeEn = true;
      measurementActive=true;
    state WAIT_END
      entry:
      writeEn= false;
    state SET_MODE
      entry:
      writeMsg = buildMode3Msg();
      writeEn = true;
    state WAIT_MODE
      entry:
      writeEn = false;
    state WRITE_P1
      entry:
      writeMsg = buildTargetMsg( ...
      426.9750, 54.0223, 574.0360, ...
      90.0000, 89.0000, 90.0000, ...
      2, 35);
      writeEn = true;
    state START_MOVE
      entry:
      writeMsg = buildEndFalseMsg();
      writeEn = true;
    state WAIT_P1
      entry:
      writeEn = false;
    state SEND_POLL
      entry:
      writeMsg=buildPosReadFrame();
      writeEn=true;
    state HOLD
      entry:
      writeEn = false;
      measurementActive=false;
    state WRITE_P2
      entry:
      writeMsg = buildTargetMsg( ...
      420.1710, -93.1800, 574.0360, ...
      70.2850, 89.0000, 90.0000, ...
      2, 42);
      writeEn = true;
    state WAIT_P2
      entry:
      writeEn = false;
    state WAIT_POLL
      entry:
      writeEn=false;
    state WRITE_P3
      entry:
      writeMsg = buildTargetMsg( ...
      466.6860, -109.8400, 443.9820, ...
      156.8940, 72.8388, 176.7590, ...
      2, 42);
      writeEn = true;
    state WAIT_P3
      entry:
      writeEn = false;
    state WRITE_P4
      entry:
      writeMsg = buildTargetMsg( ...
      477.7830, 39.8285, 443.9820, ...
      174.9040, 72.8388, 176.7590, ...
      2, 42);
      writeEn = true;
    state WAIT_P4
      entry:
      writeEn = false
    state WRITE_P5
      entry:
      writeMsg = buildTargetMsg( ...
      426.9750, 54.0223, 574.0360, ...
      90.0000, 89.0000, 90.0000, ...
      2, 42);
      writeEn = true;
    state WAIT_P5
      entry:
      writeEn = false
    state STOP_MOVE
      entry:
      writeMsg = buildEndTrueMsg();
      writeEn = true;
    (default) -> IDLE
    HOLD -> IDLE : [~startButton]
    IDLE -> INIT_END : [startButton]
    INIT_END -> WAIT_END : after(1,tick)
    WAIT_END -> SET_MODE : after(30,tick)
    SET_MODE -> WAIT_MODE : after(1,tick)
    WAIT_MODE -> WRITE_P1 : [after(30,tick)]
    WRITE_P1 -> START_MOVE : after(1,tick)
    WAIT_P1 -> SEND_POLL : after(1,tick)
    START_MOVE -> WAIT_P1 : after(1,tick)
    SEND_POLL -> WAIT_POLL : after(1,tick)
    STOP_MOVE -> HOLD : after(1,tick)
    WRITE_P2 -> WAIT_P2 : after(1,tick)
    WAIT_POLL -> WRITE_P2 : after(10,tick)
    WAIT_P2 -> WRITE_P3 : after(10,tick)
    WRITE_P3 -> WAIT_P3 : after(1,tick)
    WAIT_P3 -> WRITE_P4 : after(10,tick)
    WRITE_P4 -> WAIT_P4 : after(1,tick)
    WAIT_P4 -> WRITE_P5 : after(10,tick)
    WRITE_P5 -> WAIT_P5 : after(1,tick)
    WAIT_P5 -> STOP_MOVE : after(10,tick)
  data: msg function_output; msg function_output; msg function_output; x function_input; y function_input; z function_input; a function_input; b function_input; c function_input; s function_input; t function_input; msg function_output; msg function_output; msgKeyZminus constant uint8 size=[1 21] =uint8([0,5,0,14,1,0,7,uint8('KEYFLAG'),0,2,uint8('05'),0,0,0]); msgKeyZplus constant uint8 size=[1 21] =uint8([0,6,0,14,1,0,7,uint8('KEYFLAG'),0,2,uint8('06'),0,0,0]); msgKey0 constant uint8 size=[1 21] =uint8([0,21,0,13,1,0,7,uint8('KEYFLAG'),0,1,uint8('0'),0,0,0,0]); msgActOn constant uint8 size=[1 21] =uint8([0,60,0,16,1,0,7,uint8('ACTFLAG'),0,4,uint8('TRUE'),0]); msgActOff constant uint8 size=[1 21] =uint8([0,60,0,17,1,0,7,uint8('ACTFLAG'),0,5,uint8('FALSE')]); activeKey local uint8 =0; prevZplus local boolean size=[1]; prevZminus local boolean size=[1]; startButton input; fallActive local boolean size=[1]; riseZminus local boolean size=[1]; riseZplus local boolean size=[1]; writeMsg output uint8 size=[1 256]; writeEn output; data local; data1 local; measurementActive output; respData input uint8; curY local double; curZ local double; curX local double; TOL local double =2.0; newData input boolean
  function msg= buildEndTrueMsg:
    | function msg= buildEndTrueMsg()
    | 
    | msg = uint8([0,20, ...
    |     0,16, 1,0,7, uint8('ENDPROG'), 0,4 , uint8('TRUE')]);
    | 
    | end
  function msg = buildMode3Msg:
    | function msg = buildMode3Msg()
    | 
    | progmsg = uint8([ ...
    |     0,30, ...
    |     0,13, ...
    |     1, ...
    |     0,7, ...
    |     uint8('PROGVAR'), ...
    |     0,1, ...
    |     uint8('3')]);
    | 
    | actmsg = uint8([ ...
    |     0,60, ...
    |     0,16, ...
    |     1, ...
    |     0,7, ...
    |     uint8('ACTFLAG'), ...
    |     0,4, ...
    |     uint8('TRUE')]);
    | 
    | endmsg = uint8([ ...
    |     0,20, ...
    |     0,16, ...
    |     1, ...
    |     0,7, ...
    |     uint8('ENDPROG'), ...
    |     0,4, ...
    |     uint8('TRUE')]);
    | 
    | msg = [progmsg, actmsg, endmsg];
    | 
    | end
  function msg = buildTargetMsg(x,y,z,a,b,c,s,t):
    | function msg = buildTargetMsg(x,y,z,a,b,c,s,t)
    | 
    | s = int32(s);
    | t = int32(t);
    | 
    | tempChar = sprintf( ...
    |     '{POS: X %.1f,Y %.1f,Z %.1f,A %.1f,B %.1f,C %.1f,S %d,T %d}', ...
    |     x,y,z,a,b,c,s,t);
    | 
    | temp = uint8(tempChar);
    | 
    | msg = uint8([ ...
    |     0,13, ...
    |     0,3+8+length(temp)+2, ...
    |     1, ...
    |     0,8, ...
    |     uint8('MAT_POS1'), ...
    |     0,length(temp), ...
    |     temp]);
    | 
    | end
  function msg = buildEndFalseMsg:
    | function msg = buildEndFalseMsg()
    | 
    | msg = uint8([0,20 ,0 ,17,1,0,7,uint8('ENDPROG'),0,5,uint8('FALSE')]);
    | 
    | end
  function msg = buildPosReadFrame:
    | function msg = buildPosReadFrame()
    |     % reine $POS_ACT-Leseanfrage, ohne FINISH1/2
    |     msg = uint8([0,74,0,3+8,0,0,8,uint8('$POS_ACT')]);
    | end

== matlab function SuR_Projekt_Wegpunkt_v3/MATLAB Function2 ==
  data: data input; X output; Y output; Z output; A output; B output; C output
function [X,Y,Z,A,B,C] = fcn(data)

% Standardwerte
X = NaN;
Y = NaN;
Z = NaN;
A = NaN;
B = NaN;
C = NaN;

% Empfangsdaten in einen Vektor umwandeln
data = data(:);

% Positionen suchen
ix = find(data == 88, 1, 'first');   % X
iy = find(data == 89, 1, 'first');   % Y
iz = find(data == 90, 1, 'first');   % Z
ia = find(data == 65, 1, 'first');   % A
ib = find(data == 66, 1, 'first');   % B
ic = find(data == 67, 1, 'first');   % C

% Zahlen auslesen
if ~isempty(ix)
    X = parseNumber(data, ix + 1);
end

if ~isempty(iy)
    Y = parseNumber(data, iy + 1);
end

if ~isempty(iz)
    Z = parseNumber(data, iz + 1);
end

if ~isempty(ia)
    A = parseNumber(data, ia + 1);
end

if ~isempty(ib)
    B = parseNumber(data, ib + 1);
end

if ~isempty(ic)
    C = parseNumber(data, ic + 1);
end

end


function value = parseNumber(data, startIndex)

value = 0;

n = numel(data);
idx = startIndex;

% Sicherstellen, dass idx ein Skalar ist
idx = idx(1);

% Leerzeichen überspringen
while idx <= n
    if data(idx) ~= 32
        break;
    end
    idx = idx + 1;
end

% Vorzeichen
sgn = 1;

if idx <= n
    if data(idx) == 45       % '-'
        sgn = -1;
        idx = idx + 1;
    elseif data(idx) == 43   % '+'
        idx = idx + 1;
    end
end

% Ganzzahlteil
while idx <= n
    if data(idx) < 48 || data(idx) > 57
        break;
    end

    value = value * 10 + double(data(idx) - 48);
    idx = idx + 1;
end

% Nachkommastellen
if idx <= n && data(idx) == 46       % '.'
    idx = idx + 1;

    factor = 0.1;

    while idx <= n
        if data(idx) < 48 || data(idx) > 57
            break;
        end

        value = value + double(data(idx) - 48) * factor;
        factor = factor * 0.1;
        idx = idx + 1;
    end
end

value = sgn * value;

end
